simulink model "mpc_genC"  (R2017a)
settings: Solver=FixedStepAuto  StartTime=0.0  StopTime=10.0  FixedStep=1e-6  RelTol=1e-3
libraries: mpclib x1
settings Model: Creator=carma  LastModifiedBy=carma
settings OptimizationCC: DefaultParameterBehavior=Inlined  PassReuseOutputArgsAs=Individual arguments
settings DebuggingCC: ParameterTunabilityLossMsg=error
settings SFSimCC: MATLABDynamicMemAlloc=off
settings RTWCC: SystemTargetFile=ert.tlc  TemplateMakefile=ert_default_tmf  Description=Embedded Coder  GenerateReport=on  IncludeHyperlinkInReport=on  LaunchReport=on  GenerateTraceInfo=on  GenerateTraceReport=on  GenerateTraceReportSl=on  GenerateTraceReportSf=on  GenerateTraceReportEml=on
settings CodeAppCC: ForceParamTrailComments=on  IgnoreCustomStorageClasses=off  OperatorAnnotations=on  SimulinkDataObjDesc=on  SFDataObjDesc=on  MATLABFcnDesc=on  InsertBlockDesc=on  MATLABSourceComments=on
settings ERTTargetCC: TargetLangStandard=C99 (ISO)  GenerateSampleERTMain=on  InlinedParameterPlacement=NonHierarchical  ERTCustomFileTemplate=example_file_process.tlc

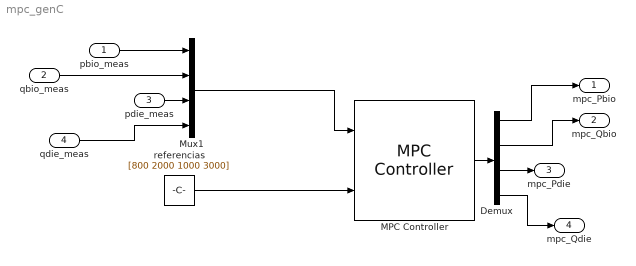
== system mpc_genC ==
  pbio_meas : Inport
  qbio_meas : Inport  Port=2
  pdie_meas : Inport  Port=3
  qdie_meas : Inport  Port=4
  Demux : Demux
  MPC Controller : mpclib/MPC Controller  SCDEnableBlockLinearizationSpecification=on  mpcobj=mpcobj  is_multiple=0  enable_value=0  return_u0=off  ref_from_ws=off  ref_signal_name=[]  ref_preview=off  md_from_ws=off  md_signal_name=[]  md_preview=off  from_project=off  project_file=MPCtask.mat  md_inport=off  mv_inport=off  cost_outport=off  return_sequence=off  return_qpstatus=off  return_state=off  state_inport=off  lims_inport=off  ywt_inport=off  is_designfromscratch=0  uwt_inport=off  duwt_inport=off  rhoeps_inport=off  uref_inport=off  n_ts=0.03  n_mv=4  n_md=0  n_ud=0  n_mo=4  n_uo=0  BlockDataType=double  SampleTimeInherited=off  switch_inport=off
  Mux1 : Mux
  referencias : Constant  Value=[800 2000 1000 3000]
  mpc_Pbio : Outport
  mpc_Qbio : Outport  Port=2
  mpc_Pdie : Outport  Port=3
  mpc_Qdie : Outport  Port=4
  wires:
  Mux1/1 -> MPC Controller/1
  pdie_meas/1 -> Mux1/3
  qdie_meas/1 -> Mux1/4
  Demux/1 -> mpc_Pbio/1
  MPC Controller/1 -> Demux/1
  qbio_meas/1 -> Mux1/2
  Demux/3 -> mpc_Pdie/1
  pbio_meas/1 -> Mux1/1
  Demux/2 -> mpc_Qbio/1
  Demux/4 -> mpc_Qdie/1
  referencias/1 -> MPC Controller/2
